simulink model "BipedWalking_3D"  (R2019b)
settings: Solver=VariableStepAuto  StartTime=0.0  StopTime=100  RelTol=1e-3  EnableMultiTasking=on
undefined symbols (not defined in the file or in its folder): X, Y, Z
libraries: sm_lib x50, nesl_utility x32, Contact_Forces_Lib x8, walkingRobotUtils x1
(part 3 of 3)

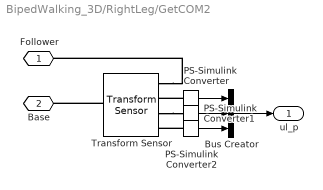
== system BipedWalking_3D/RightLeg/GetCOM2 ==
  Bus Creator : BusCreator  Inputs=3
  PS-Simulink Converter : nesl_utility/PS-Simulink Converter  PhysicalDomain=network_engine_domain  SubClassName=ps_output  LeftPortType=input  RightPortType=output  PseudoPeriodic=off  Frequencies=[]  Unit=cm  AffineConversion=off
  PS-Simulink Converter1 : nesl_utility/PS-Simulink Converter  PhysicalDomain=network_engine_domain  SubClassName=ps_output  LeftPortType=input  RightPortType=output  PseudoPeriodic=off  Frequencies=[]  Unit=cm  AffineConversion=off
  PS-Simulink Converter2 : nesl_utility/PS-Simulink Converter  PhysicalDomain=network_engine_domain  SubClassName=ps_output  LeftPortType=input  RightPortType=output  PseudoPeriodic=off  Frequencies=[]  Unit=cm  AffineConversion=off
  Transform Sensor : sm_lib/Frames and Transforms/Transform Sensor  MeasurementFrame=World  SenseAngle=off  SenseAxis=off  SenseAngle1=off  SenseAngle2=off  SenseAngle3=off  SenseQ=off  SenseR=off  SenseOmegaX=off  SenseOmegaY=off  SenseOmegaZ=off  SenseOmega1=off  SenseOmega2=off  SenseOmega3=off  SenseQDot=off  SenseRDot=off  SenseAlphaX=off  SenseAlphaY=off  SenseAlphaZ=off  SenseAlpha1=off  SenseAlpha2=off  SenseAlpha3=off  SenseQDDot=off  SenseRDDot=off  SenseX=on  SenseY=on  SenseZ=on  SenseRad=off  SenseAzim=off  SenseDist=off  SenseInc=off  SenseXDot=off  SenseYDot=off  SenseZDot=off  SenseRadDot=off  SenseAzimDot=off  SenseDistDot=off  SenseIncDot=off  SenseXDDot=off  SenseYDDot=off  SenseZDDot=off  SenseRadDDot=off  SenseAzimDDot=off  SenseDistDDot=off  SenseIncDDot=off
  Follower : PMIOPort  Side=Right
  Base : PMIOPort  Port=2  Side=Left
  "ul_p " : Outport
  wires:
  Bus Creator/1 -> "ul_p "/1
  PS-Simulink Converter/1 -> Bus Creator/1
  PS-Simulink Converter1/1 -> Bus Creator/2
  PS-Simulink Converter2/1 -> Bus Creator/3
  connections:
  Transform Sensor/RConn1 -- Follower/RConn1
  Transform Sensor/LConn1 -- Base/RConn1
  PS-Simulink Converter/LConn1 -- Transform Sensor/RConn2
  PS-Simulink Converter2/LConn1 -- Transform Sensor/RConn4
  Transform Sensor/RConn3 -- PS-Simulink Converter1/LConn1

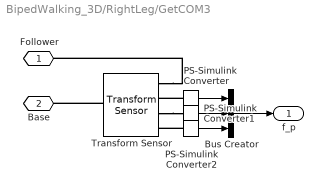
== system BipedWalking_3D/RightLeg/GetCOM3 ==
  Bus Creator : BusCreator  Inputs=3
  PS-Simulink Converter : nesl_utility/PS-Simulink Converter  PhysicalDomain=network_engine_domain  SubClassName=ps_output  LeftPortType=input  RightPortType=output  PseudoPeriodic=off  Frequencies=[]  Unit=cm  AffineConversion=off
  PS-Simulink Converter1 : nesl_utility/PS-Simulink Converter  PhysicalDomain=network_engine_domain  SubClassName=ps_output  LeftPortType=input  RightPortType=output  PseudoPeriodic=off  Frequencies=[]  Unit=cm  AffineConversion=off
  PS-Simulink Converter2 : nesl_utility/PS-Simulink Converter  PhysicalDomain=network_engine_domain  SubClassName=ps_output  LeftPortType=input  RightPortType=output  PseudoPeriodic=off  Frequencies=[]  Unit=cm  AffineConversion=off
  Transform Sensor : sm_lib/Frames and Transforms/Transform Sensor  MeasurementFrame=World  SenseAngle=off  SenseAxis=off  SenseAngle1=off  SenseAngle2=off  SenseAngle3=off  SenseQ=off  SenseR=off  SenseOmegaX=off  SenseOmegaY=off  SenseOmegaZ=off  SenseOmega1=off  SenseOmega2=off  SenseOmega3=off  SenseQDot=off  SenseRDot=off  SenseAlphaX=off  SenseAlphaY=off  SenseAlphaZ=off  SenseAlpha1=off  SenseAlpha2=off  SenseAlpha3=off  SenseQDDot=off  SenseRDDot=off  SenseX=on  SenseY=on  SenseZ=on  SenseRad=off  SenseAzim=off  SenseDist=off  SenseInc=off  SenseXDot=off  SenseYDot=off  SenseZDot=off  SenseRadDot=off  SenseAzimDot=off  SenseDistDot=off  SenseIncDot=off  SenseXDDot=off  SenseYDDot=off  SenseZDDot=off  SenseRadDDot=off  SenseAzimDDot=off  SenseDistDDot=off  SenseIncDDot=off
  Follower : PMIOPort  Side=Right
  Base : PMIOPort  Port=2  Side=Left
  "f_p " : Outport
  wires:
  Bus Creator/1 -> "f_p "/1
  PS-Simulink Converter/1 -> Bus Creator/1
  PS-Simulink Converter1/1 -> Bus Creator/2
  PS-Simulink Converter2/1 -> Bus Creator/3
  connections:
  Transform Sensor/RConn1 -- Follower/RConn1
  Transform Sensor/LConn1 -- Base/RConn1
  PS-Simulink Converter/LConn1 -- Transform Sensor/RConn2
  PS-Simulink Converter2/LConn1 -- Transform Sensor/RConn4
  Transform Sensor/RConn3 -- PS-Simulink Converter1/LConn1

== matlab function BipedWalking_3D/LeftLeg/MATLAB Function ==
  data: ul_x input; com_x output; ul_y input; ul_z input; com_y output; com_z output; ll_x input; ll_y input; ll_z input; f_x input; f_y input; f_z input
function [com_x,com_y,com_z] = COM(ul_x, ul_y, ul_z, ll_x, ll_y, ll_z, f_x, f_y, f_z)
    ul_m = 0.314159;
    ll_m = 0.314159;
    f_m = 0.3;
    
com_x = (ul_m*ul_x + ll_m*ll_x + f_m*f_x)/(ul_m + ll_m + f_m);
com_y = (ul_m*ul_y + ll_m*ll_y + f_m*f_y)/(ul_m + ll_m + f_m);
com_z = (ul_m*ul_z + ll_m*ll_z + f_m*f_z)/(ul_m + ll_m + f_m);

== matlab function BipedWalking_3D/RightLeg/MATLAB Function ==
  data: ul_x input; com_x output; ul_y input; ul_z input; com_y output; com_z output; ll_x input; ll_y input; ll_z input; f_x input; f_y input; f_z input
function [com_x,com_y,com_z] = COM(ul_x, ul_y, ul_z, ll_x, ll_y, ll_z, f_x, f_y, f_z)
    ul_m = 0.314159;
    ll_m = 0.314159;
    f_m = 0.3;
    
com_x = (ul_m*ul_x + ll_m*ll_x + f_m*f_x)/(ul_m + ll_m + f_m);
com_y = (ul_m*ul_y + ll_m*ll_y + f_m*f_y)/(ul_m + ll_m + f_m);
com_z = (ul_m*ul_z + ll_m*ll_z + f_m*f_z)/(ul_m + ll_m + f_m);

== matlab function BipedWalking_3D/MATLAB Function ==
  data: l_x input; com_x output; l_y input; l_z input; com_y output; com_z output; r_x input; r_y input; r_z input; t_x input; t_y input; t_z input
function [com_x,com_y,com_z] = COM(l_x, l_y, l_z, r_x, r_y, r_z, t_x, t_y, t_z)
    r = 0.928318;
    l = 0.928318;
    t = 9;
    
com_x = (r*r_x + l*l_x + t*t_x)/(r + l + t);
com_y = (r*r_y + l*l_y + t*t_y)/(r + l + t);
com_z = (r*r_z + l*l_z + t*t_z)/(r + l + t);
